simulink model "FIR_referenced"  (R2020b)
settings: Solver=FixedStepDiscrete  StartTime=0.0  StopTime=1  FixedStep=0.001  RelTol=1e-3
settings Model: Creator=abhin  LastModifiedBy=abhin
settings DataIOCC: SaveOutput=off  SaveTime=off

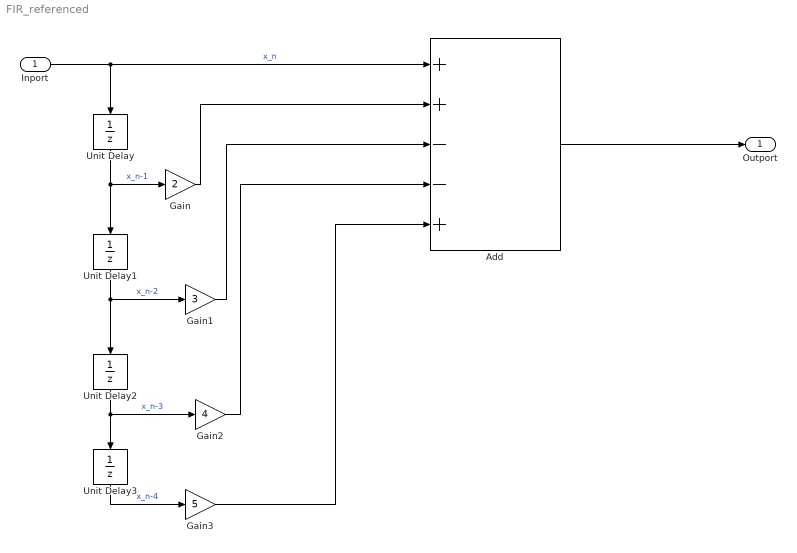
== system FIR_referenced ==
  Inport : Inport  OutDataTypeStr=double  PortDimensions=1  SampleTime=[0.001,0]
  Add : Sum  Inputs=++--+
  Gain : Gain  Gain=2
  Gain1 : Gain  Gain=3
  Gain2 : Gain  Gain=4
  Gain3 : Gain  Gain=5
  Unit Delay{,1..3} (4 alike) : UnitDelay  SampleTime=-1  HasFrameUpgradeWarning=on
  Outport : Outport  OutDataTypeStr=double  PortDimensions=1  SampleTime=[0.001,0]
  wires:
  Inport/1 -> Unit Delay/1, Add/1  "x_n"
  Add/1 -> Outport/1
  Unit Delay1/1 -> Unit Delay2/1, Gain1/1  "x_n-2"
  Gain3/1 -> Add/5
  Unit Delay2/1 -> Gain2/1, Unit Delay3/1  "x_n-3"
  Gain2/1 -> Add/4
  Unit Delay3/1 -> Gain3/1  "x_n-4"
  Gain/1 -> Add/2
  Unit Delay/1 -> Gain/1, Unit Delay1/1  "x_n-1"
  Gain1/1 -> Add/3
